simulink model "simo"  (Simulink 2.20)
settings: Solver=ode45  StartTime=0.0  StopTime=20  MaxStep=10  RelTol=1e-3  AbsTol=1e-6
settings Model: ExternalInput=[]  SaveTime=off  SaveOutput=off  InitialState=[]  ConsistencyChecking=off  RTWPlaceOutputsASAP=off  RTWLocalBlockOutputs=on

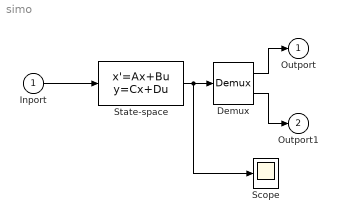
== system simo ==
  Inport : Inport  Port=1  PortWidth=-1  SampleTime=-1
  Demux : Demux  Outputs=2
  Scope : Scope
      settings: TickLabels=on  TimeRange=20  YMin=-2  YMax=6  SaveToWorkspace=off  SaveName=ScopeData
  State-space : StateSpace  A=[-0.3 0 0;2.9 -0.62,-2.3;0,2.3,0]  B=[1;0;0]  C=[1 1 0; 1 -3 1]  D=[0;1]  X0=[1;1;1]
  Outport : Outport  Port=1  InitialOutput=0
  Outport1 : Outport  Port=2  InitialOutput=0
  wires:
  State-space/1 -> Scope/1, Demux/1
  Inport/1 -> State-space/1
  Demux/1 -> Outport/1
  Demux/2 -> Outport1/1
